simulink model "model"  (R2021a)
settings: Solver=VariableStepAuto  StartTime=0.0  StopTime=86400  RelTol=1e-3
undefined symbols (not defined in the file): Ion, Lithium
libraries: spsControlledCurrentSourceLib x2, spsIdealSwitchLib x2, spsSeriesRLCBranchLib x2, spsBatteryLib x1, spsGroundLib x1, spspowerguiLib x1
settings Model: Creator=S288338  LastModifiedBy=Administrator
settings SolverCC: AlgebraicLoopSolver=TrustRegion
settings DebuggingCC: SFMachineParentedDataDiag=warning

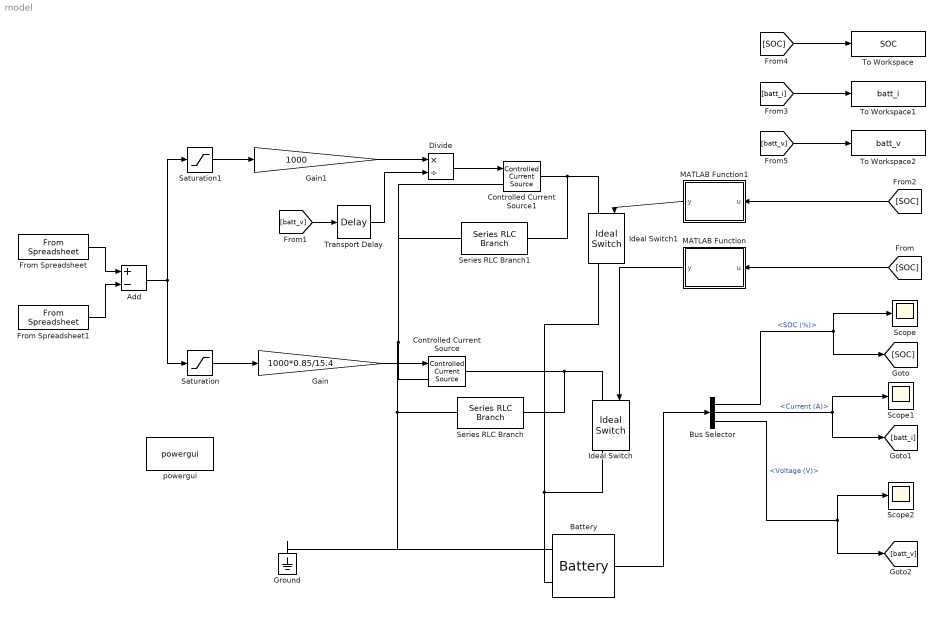
== system model ==
  Add : Sum  Inputs=+-
  Battery : spsBatteryLib/Battery  BatType=Lithium-Ion  ShowTempParam=off  ThermalPreset=no  ShowAgeParam=off  NomV=15.4  NomQ=856  SOC=30  Batt_Tr=1  PresetModel=on  MaxQ=856  MinV=11.55  FullV=17.9254  Dis_rate=372.1739  R=0.00017991  Normal_OP=774.1217  expZone="[16.6379      42.0557]"  current=[6.5 13 32.5]  Units=Time  Tci=20  NomT=20  T2=-30  MaxQ2=4.8  FullV2=7.1  Normal_OP2=5.655  expZone2="[6.58           1]"  Rca=0.6  ti=2000  Dp=0  Neq0=0  Tsim=1e6  Ta1=25  Qeol=5.4*0.9  Reol=0.013333*1.2  Char_age=[2.3478, 3]  Dis_age=[2.3478, 10]  N1=1500  N2=10500  N3=1000  N4=1400  Ta2=45  N5=950
  Bus Selector : BusSelector  OutputSignals=SOC (%),Current (A),Voltage (V)
  Controlled Current Source : spsControlledCurrentSourceLib/Controlled Current Source  Initialize=off  Source_Type=AC  Amplitude=0  Phase=0  Frequency=0  Measurements=None
  Controlled Current Source1 : spsControlledCurrentSourceLib/Controlled Current Source  Initialize=off  Source_Type=AC  Amplitude=0  Phase=0  Frequency=0  Measurements=None
  Divide : Product  Inputs=*/
  From Spreadsheet : FromSpreadsheet  FileName=input.xlsx  SheetName=PV1
  From Spreadsheet1 : FromSpreadsheet  FileName=input.xlsx  SheetName=House1
  Gain : Gain  Gain=1000*0.85/15.4
  Gain1 : Gain  Gain=1000
  Ground : spsGroundLib/Ground  LConnTagsString=a
  Ideal Switch : spsIdealSwitchLib/Ideal Switch  Ron=0.001  Lon=0  IC=0  Rs=inf  Cs=inf  Measurements=on
  Ideal Switch1 : spsIdealSwitchLib/Ideal Switch  Ron=0.001  Lon=0  IC=0  Rs=inf  Cs=inf  Measurements=on
  MATLAB Function : MATLAB Function  TreatAsAtomicUnit=on
  MATLAB Function1 : MATLAB Function  TreatAsAtomicUnit=on
  Saturation : Saturate  UpperLimit=inf  LowerLimit=0
  Saturation1 : Saturate  UpperLimit=0  LowerLimit=-inf
  Scope : Scope
  Scope1 : Scope
  Scope2 : Scope
  Series RLC Branch : spsSeriesRLCBranchLib/Series RLC Branch  LConnTagsString=__new0  RConnTagsString=__new0  BranchType=R  Resistance=1E8  Inductance=1e-3  SetiL0=off  InitialCurrent=0  Capacitance=1e-6  Setx0=off  InitialVoltage=0  Measurements=None
  Series RLC Branch1 : spsSeriesRLCBranchLib/Series RLC Branch  LConnTagsString=__new0  RConnTagsString=__new0  BranchType=R  Resistance=1E8  Inductance=1e-3  SetiL0=off  InitialCurrent=0  Capacitance=1e-6  Setx0=off  InitialVoltage=0  Measurements=None
  To Workspace : ToWorkspace  VariableName=SOC  SaveFormat=Timeseries  SampleTime=-1
  To Workspace1 : ToWorkspace  VariableName=batt_i  SaveFormat=Timeseries  SampleTime=-1
  To Workspace2 : ToWorkspace  VariableName=batt_v  SaveFormat=Timeseries  SampleTime=-1
  Transport Delay : TransportDelay  InitialOutput=15.4
  powergui : spspowerguiLib/powergui  Priority=1  SimulationMode=Continuous  SampleTime=50e-6  frequency=60  Iterations=50  frequencyindice=0  Pbase=100e6  ErrMax=1e-4  UnitsV=kV  UnitsW=MW  buscounter=0  FunctionMessages=off  echomessages=off  EnableUseOfTLC=off  CurrentSourceSwitches=off  DisableSnubberDevices=off  DisableRonSwitches=off  DisableVfSwitches=off  DisplayEquations=off  AutomaticDiscreteSolvers=off  SolverType=Tustin/Backward Euler (TBE)  Interpol=off  ExternalGateDelay=off  methode=off  Ts=100  x0status=blocks  SPID=on  SwTol=0  HookPort=off  NonlinearTolerance=1e-4  nMaxIteration=100  ContinueOnMaxIteration=off  RestoreLinks=warning  ResistiveCurrentMeasurement=off  Frange=[0:2:500]  Ylog=off  Xlog=on  ShowGrid=off  save=off  variable=ZData  structure=0  ZoomFFT=off  StartTime=0.0  cycles=1  DisplayStyle=1  fundamental=60  FreqAxis=off  MaxFrequency=1000  frequencyindicesteady=1  RmsSteady=1  display=off
  wires:
  From Spreadsheet/1 -> Add/1
  From Spreadsheet1/1 -> Add/2
  Add/1 -> Saturation/1, Saturation1/1
  Saturation/1 -> Gain/1
  Gain/1 -> Controlled Current Source/1
  Battery/1 -> Bus Selector/1
  Bus Selector/1 -> [SOC], Scope/1  "<SOC (%)>"
  Bus Selector/2 -> [batt_i], Scope1/1  "<Current (A)>"
  Bus Selector/3 -> [batt_v], Scope2/1  "<Voltage (V)>"
  [SOC] -> MATLAB Function/1(u)
  MATLAB Function/1(y) -> Ideal Switch/1
  Saturation1/1 -> Gain1/1
  Gain1/1 -> Divide/1
  Transport Delay/1 -> Divide/2
  [batt_v] -> Transport Delay/1
  Divide/1 -> Controlled Current Source1/1
  [SOC] -> MATLAB Function1/1(u)
  MATLAB Function1/1(y) -> Ideal Switch1/1
  [batt_v] -> To Workspace2/1
  [batt_i] -> To Workspace1/1
  [SOC] -> To Workspace/1
  connections:
  Controlled Current Source/RConn1 -- Series RLC Branch/RConn1 -- Ideal Switch/LConn1
  Ideal Switch/RConn1 -- Battery/LConn1 -- Ideal Switch1/RConn1
  Controlled Current Source/LConn1 -- Series RLC Branch1/LConn1 -- Controlled Current Source1/LConn1 -- Ground/LConn1 -- Battery/LConn2 -- Series RLC Branch/LConn1
  Controlled Current Source1/RConn1 -- Series RLC Branch1/RConn1 -- Ideal Switch1/LConn1

== matlab function model/MATLAB Function ==
  data: u input; y output
function y = fcn(u)

if u>99
    y=0;

else 
    y=1;

end
end

== matlab function model/MATLAB Function1 ==
  data: u input; y output
function y = fcn(u)

if u<10
    y=0;

else 
    y=1;

end
end
